simulink model "stateflow_atomic_subchart"  (Simulink 8.6)
settings: Solver=VariableStepAuto  StartTime=0.0  StopTime=10.0  RelTol=1e-3
settings Model: Creator=ladmin  LastModifiedBy=ladmin
settings DataIOCC: SaveFormat=Dataset  SignalLoggingSaveFormat=Dataset
settings OptimizationCC: ExpressionDepthLimit=128
settings DebuggingCC: UnderspecifiedInitializationDetection=Simplified  MergeDetectMultiDrivingBlocksExec=error  SolverPrmCheckMsg=none  FcnCallInpInsideContextMsg=EnableAllAsError  StateNameClashWarn=none
settings HardwareCC: ProdBitPerPointer=64  ProdLargestAtomicFloat=Float  ProdIntDivRoundTo=Zero  ProdEndianess=LittleEndian  ProdWordSize=64  ProdHWDeviceType=Intel->x86-64 (Windows64)
settings GRTTargetCC: GeneratePreprocessorConditionals=Use local settings  CombineOutputUpdateFcns=on  GRTInterface=off
settings ConfigComp: CovModelRefEnable=off

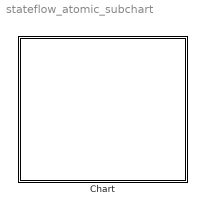
== system stateflow_atomic_subchart ==
  Chart : Stateflow chart  TreatAsAtomicUnit=on

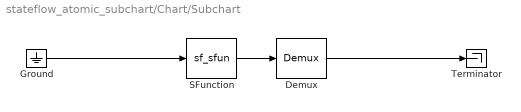
== system stateflow_atomic_subchart/Chart/Subchart ==
  " Demux " : Demux  Outputs=1
  " Ground " : Ground
  " SFunction " : S-Function  Tag=Stateflow S-Function stateflow_atomic_subchart 1  FunctionName=sf_sfun  PortCounts=[1 1]  SFunctionDeploymentMode=off  EnableBusSupport=off
  " Terminator " : Terminator
  wires:
  " Ground "/1 -> " SFunction "/1
  " Demux "/1 -> " Terminator "/1
  " SFunction "/1 -> " Demux "/1

== stateflow chart Chart/Subchart ==
  state State_lvl2_1
  state State_lvl2_2
  State_lvl2_1 -> State_lvl2_2

== stateflow chart Chart ==
  state State_lvl1
  state Subchart
